simulink model "ModelHeatTreatment"  (R2020b)
settings: Solver=FixedStepAuto  StartTime=0.0  StopTime=Inf  FixedStep=0.010  RelTol=1e-3
settings Model: Creator=kaebi  LastModifiedBy=kaebi
settings OptimizationCC: DefaultParameterBehavior=Inlined  LocalBlockOutputs=off
settings RTWCC: Description=TwinCAT GRT Target  SystemTargetFile=TwinCatGrt.tlc  GenCodeOnly=on  TemplateMakefile=tcgrt_msbuild.tmf  TargetLang=C++
settings STFCustomTargetCC: TargetLangStandard=C++03 (ISO)  ConcurrentExecutionCompliant=off  CombineOutputUpdateFcns=on  CodeInterfacePackaging=Reusable function  GRTInterface=off  GenerateAllocFcn=on  SystemTargetFile=TwinCatGrt.tlc
settings GRTTargetCC: TargetLangStandard=C++03 (ISO)  ParMdlRefBuildCompliant=off  CompOptLevelCompliant=off  ConcurrentExecutionCompliant=off  MatFileLogging=off  CodeInterfacePackaging=Reusable function  GenerateAllocFcn=on  UseToolchainInfoCompliant=off  ExtModeMexFile=TcExtModeClient

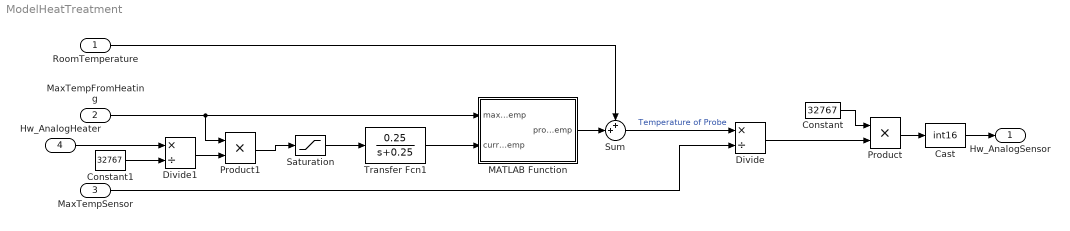
== system ModelHeatTreatment ==
  RoomTemperature : Inport
  MaxTempFromHeating : Inport  Port=2
  MaxTempSensor : Inport  Port=3
  Hw_AnalogHeater : Inport  Port=4  OutDataTypeStr=int16
  Cast : DataTypeConversion  OutDataTypeStr=int16
  Constant : Constant  Value=32767
  Constant1 : Constant  Value=32767
  Divide : Product  Inputs=*/
  Divide1 : Product  Inputs=*/  OutDataTypeStr=double
  MATLAB Function : MATLAB Function  TreatAsAtomicUnit=on
  Product : Product
  Product1 : Product
  Saturation : Saturate  UpperLimit=inf  LowerLimit=0
  Sum : Sum  Inputs=++|
  Transfer Fcn1 : TransferFcn  Numerator=[0.25]  Denominator=[1 0.25]
  Hw_AnalogSensor : Outport  OutDataTypeStr=int16
  wires:
  RoomTemperature/1 -> Sum/1
  Product/1 -> Cast/1
  Divide/1 -> Product/2
  Constant/1 -> Product/1
  Sum/1 -> Divide/1  "Temperature of Probe"
  MaxTempSensor/1 -> Divide/2
  MATLAB Function/1(probeTemp) -> Sum/2
  MaxTempFromHeating/1 -> MATLAB Function/1(maxTemp), Product1/1
  Constant1/1 -> Divide1/2
  Divide1/1 -> Product1/2
  Product1/1 -> Saturation/1
  Transfer Fcn1/1 -> MATLAB Function/2(currentTemp)
  Hw_AnalogHeater/1 -> Divide1/1
  Cast/1 -> Hw_AnalogSensor/1
  Saturation/1 -> Transfer Fcn1/1

== matlab function ModelHeatTreatment/MATLAB Function ==
  data: maxTemp input; probeTemp output; currentTemp input
function probeTemp = fcn(maxTemp, currentTemp)

if (currentTemp < 0)
    currentTemp = 0;
end

if (currentTemp > maxTemp)
    currentTemp = maxTemp;
end

probeTemp = currentTemp;
